simulink model "test"  (R2023b)
settings: Solver=FixedStepDiscrete  StartTime=0.0  StopTime=240  FixedStep=0.01  RelTol=1e-3
undefined symbols (not defined in the file or in its folder): DiscIntNeverNeededParam, InputPWM, WheelSpeed
libraries: mobileRoboticsTrainingLib x7, simulink x3
settings Model: SimulationMode=accelerator  NumberOfSteps=10  SnapshotBufferSize=20  Creator=Boitumelo  LastModifiedBy=kianf
settings DebuggingCC: UnconnectedInputMsg=warning  UnconnectedOutputMsg=warning  UnconnectedLineMsg=warning
settings ModelReferenceCC: EnableRefExpFcnMdlSchedulingChecks=on
settings RTWCC: DLArmComputeVersion=19.05

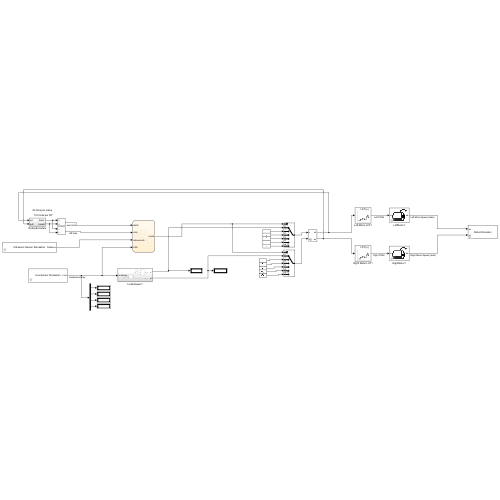
[thumbnail: Simulink's stored preview of the top-level diagram]
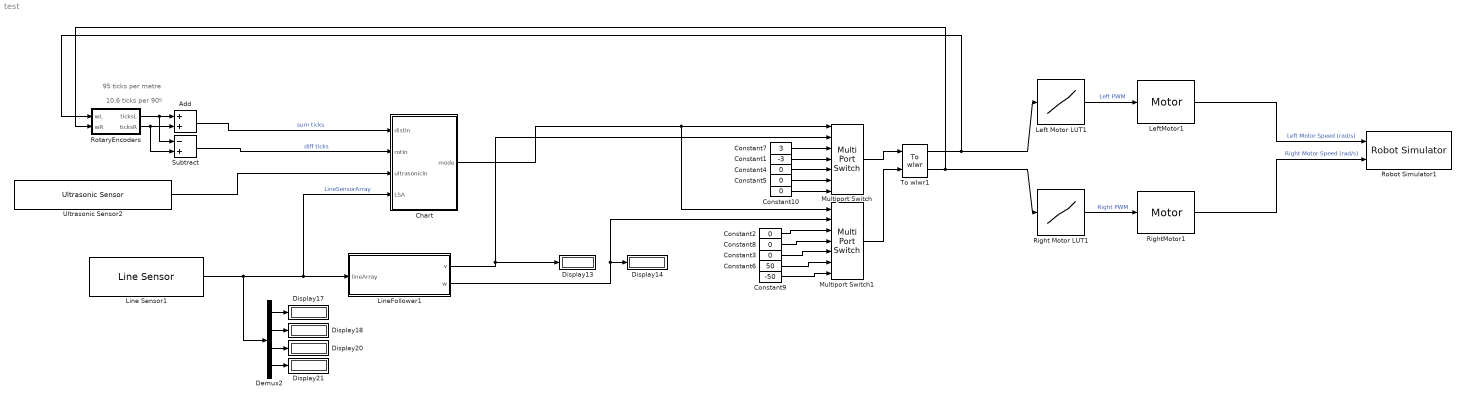
== system test ==
  note: 10.6 ticks per 90º
  note: 95 ticks per metre
  Add : Sum
  Chart : Stateflow chart  TreatAsAtomicUnit=on
  Constant1 : Constant  Value=-3
  Constant{2..5,8,10} (6 alike) : Constant  Value=0
  Constant6 : Constant  Value=50
  Constant7 : Constant  Value=3
  Constant9 : Constant  Value=-50
  Demux2 : Demux
  Display{13..14,17..18,20..21} (6 alike) : Display
  Left Motor LUT1 : Lookup_n-D  NumberOfTableDimensions=1  BreakpointsForDimension1=WheelSpeed  Table=InputPWM  InterpMethod=Nearest  ExtrapMethod=Clip  InternalRulePriority=Speed  RndMeth=Simplest
  LeftMotor1 : mobileRoboticsTrainingLib/Motor  motorPlant=wheelMotorModel  sensorType=Speed
      settings: SourceProductName=Mobile Robotics Training Library
  Line Sensor1 : mobileRoboticsTrainingLib/Line Sensor  mapVariable=mapForSim  envVal=1  lineVal=0  sensOff=[64.3e-3 35.4e-3;67.5e-3 5e-3;67.5e-3 -5e-3;64.3e-3 -35.4e-3]
      settings: SourceProductName=Mobile Robotics Training Library
  LineFollower1 : Subsystem
  Multiport Switch : MultiPortSwitch  DataPortOrder=Zero-based contiguous  Inputs=6  DataPortIndices={0,1,3,4}  zeroidx=on  SaturateOnIntegerOverflow=off
  Multiport Switch1 : MultiPortSwitch  DataPortOrder=Zero-based contiguous  Inputs=6  DataPortIndices={0,1,3,4}  zeroidx=on  SaturateOnIntegerOverflow=off  InputSameDT=off
  Right Motor LUT1 : Lookup_n-D  NumberOfTableDimensions=1  BreakpointsForDimension1=WheelSpeed  Table=InputPWM  InterpMethod=Nearest  ExtrapMethod=Clip  InternalRulePriority=Speed  RndMeth=Simplest
  RightMotor1 : mobileRoboticsTrainingLib/Motor  motorPlant=wheelMotorModel  sensorType=Speed
      settings: SourceProductName=Mobile Robotics Training Library
  Robot Simulator1 : mobileRoboticsTrainingLib/Robot Simulator  Priority=99  mapVar=mapForSim  startX=1  startY=0.27175  startTheta=90  axleLength=axleLength  wheelR=wheelR
  RotaryEncoders : Subsystem
  Subtract : Sum  Inputs=-+
  To wlwr1 : mobileRoboticsTrainingLib/To wlwr  axleLength=0.1  wheelR=0.05
      link override change parameters: Gain=[1 -axleLength/2;1 axleLength/2]
  Ultrasonic Sensor2 : mobileRoboticsTrainingLib/Ultrasonic Sensor  mapVar=mapForSim  maxSenRange=2  minSenRange=0.02  senRes=0.01  sensOff=[0 0]
      settings: SourceProductName=Mobile Robotics Training Library
  wires:
  RotaryEncoders/2(ticksR) -> Subtract/2, Add/2
  Ultrasonic Sensor2/1 -> Chart/3(ultrasonicIn)
  Demux2/3 -> Display20/1
  Demux2/2 -> Display18/1
  RotaryEncoders/1(ticksL) -> Subtract/1, Add/1
  Constant9/1 -> Multiport Switch1/7
  Add/1 -> Chart/1(distIn)  "sum ticks"
  Constant5/1 -> Multiport Switch/6
  Constant8/1 -> Multiport Switch1/4
  Multiport Switch/1 -> To wlwr1/1
  LineFollower1/2(w) -> Multiport Switch1/2, Display14/1
  Subtract/1 -> Chart/2(rotIn)  "diff ticks"
  Constant2/1 -> Multiport Switch1/3
  Demux2/4 -> Display21/1
  Constant1/1 -> Multiport Switch/4
  Constant4/1 -> Multiport Switch/5
  Demux2/1 -> Display17/1
  Constant7/1 -> Multiport Switch/3
  Constant3/1 -> Multiport Switch1/5
  Constant10/1 -> Multiport Switch/7
  Line Sensor1/1 -> Demux2/1, Chart/4(LSA), LineFollower1/1(lineArray)  "LineSensorArray"
  Constant6/1 -> Multiport Switch1/6
  Chart/1(mode) -> Multiport Switch1/1, Multiport Switch/1
  Multiport Switch1/1 -> To wlwr1/2
  LineFollower1/1(v) -> Display13/1, Multiport Switch/2
  LeftMotor1/1 -> Robot Simulator1/1  "Left Motor Speed (rad/s)"
  RightMotor1/1 -> Robot Simulator1/2  "Right Motor Speed (rad/s)"
  To wlwr1/1 -> RotaryEncoders/1(wL), Left Motor LUT1/1
  To wlwr1/2 -> Right Motor LUT1/1, RotaryEncoders/2(wR)
  Left Motor LUT1/1 -> LeftMotor1/1  "Left PWM"
  Right Motor LUT1/1 -> RightMotor1/1  "Right PWM"

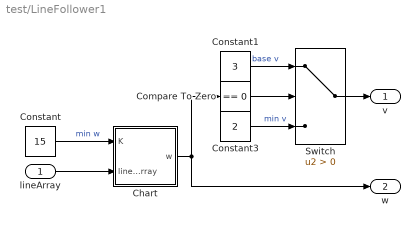
== system test/LineFollower1 ==
  lineArray : Inport
  Chart : Stateflow chart  TreatAsAtomicUnit=on
  Compare To Zero : simulink/Logic and Bit Operations/Compare To Zero  relop===  OutDataTypeStr=boolean
  Constant : Constant  Value=15
  Constant1 : Constant  Value=3
  Constant3 : Constant  Value=2
  Switch : Switch  Criteria=u2 > Threshold  SaturateOnIntegerOverflow=off  InputSameDT=off
  v : Outport
  w : Outport  Port=2
  wires:
  Constant1/1 -> Switch/1  "base v"
  Chart/1(w) -> Compare To Zero/1, w/1
  Constant3/1 -> Switch/3  "min v"
  Switch/1 -> v/1
  lineArray/1 -> Chart/2(lineArray)
  Compare To Zero/1 -> Switch/2
  Constant/1 -> Chart/1(K)  "min w"

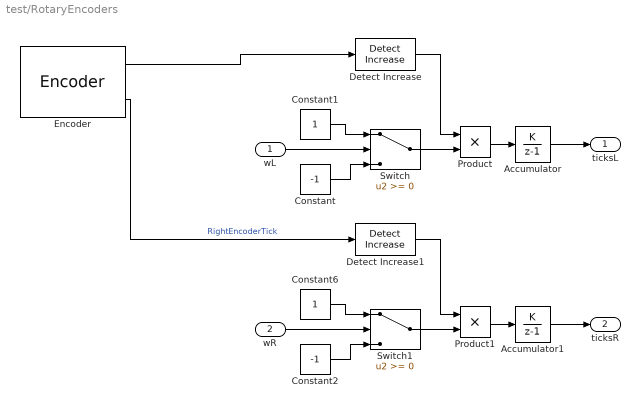
== system test/RotaryEncoders ==
  wL : Inport
  wR : Inport  Port=2
  Accumulator : DiscreteIntegrator  IntegratorMethod=Accumulation: Forward Euler  SampleTime=-1  ICPrevOutput=DiscIntNeverNeededParam  ICPrevScaledInput=DiscIntNeverNeededParam
  Accumulator1 : DiscreteIntegrator  IntegratorMethod=Accumulation: Forward Euler  SampleTime=-1  ICPrevOutput=DiscIntNeverNeededParam  ICPrevScaledInput=DiscIntNeverNeededParam
  Constant : Constant  Value=-1
  Constant1 : Constant
  Constant2 : Constant  Value=-1
  Constant6 : Constant
  Detect Increase : simulink/Logic and Bit Operations/Detect Increase  vinit=0.0  OutDataTypeStr=boolean
  Detect Increase1 : simulink/Logic and Bit Operations/Detect Increase  vinit=0.0  OutDataTypeStr=boolean
  Encoder : mobileRoboticsTrainingLib/Encoder  axleLength=axleLength  wheelR=wheelR  ticksPerRot=ticksPerRot
      settings: SourceProductName=Mobile Robotics Training Library
  Product : Product
  Product1 : Product
  Switch : Switch  SaturateOnIntegerOverflow=off  InputSameDT=off
  Switch1 : Switch  SaturateOnIntegerOverflow=off  InputSameDT=off
  ticksL : Outport
  ticksR : Outport  Port=2
  wires:
  wL/1 -> Switch/2
  Constant1/1 -> Switch/1
  Constant/1 -> Switch/3
  Encoder/1 -> Detect Increase/1
  Switch/1 -> Product/2
  Accumulator/1 -> ticksL/1
  wR/1 -> Switch1/2
  Constant6/1 -> Switch1/1
  Constant2/1 -> Switch1/3
  Accumulator1/1 -> ticksR/1
  Switch1/1 -> Product1/2
  Product/1 -> Accumulator/1
  Detect Increase/1 -> Product/1
  Detect Increase1/1 -> Product1/1
  Product1/1 -> Accumulator1/1
  Encoder/2 -> Detect Increase1/1  "RightEncoderTick"

== stateflow chart test/Chart ==
  state Setup
    entry:
    stop=0;
    objects = ones(5);
    object = 1;
  state Drive
    entry:
    mode=0;
  state DriveForward
    entry:
    mode = 1;
    distT = distIn + 8;
  state CentreOnIntersection
    entry:
    mode = 1;
    distT = distIn + 6;
  state LeftTurn
    entry:
    mode = 4;
    rotT = rotIn + 16;
  state RightTurn
    entry:
    mode = 5;
  state ErrorHandler
    entry:
    mode=4;
  state TurnAround
    entry:
    mode = 4;
    rotT = rotIn + 21;
  state ClosestObject
    entry:
    cObj = 1;
    for i = 1:5
    if objects(i) < cObj
    cObj = objects(i);
    end
    end
  state DriveBackward
    entry:
    mode = 2;
  state USmeasure
    entry:
    objects(object) = ultrasonicIn;
    object = object + 1;
  state Stop
    entry:
    mode=3;
  state Party
    state dance
      entry:
      moves = moves + 1;
    dance -> (junction 71) [order 2] : {mode=1;}
        | %1
    (junction 101) -> dance
    (junction 97) -> (junction 101) : after(125, msec)
    (junction 71) -> (junction 73) : after(250, msec)
        | {mode=2;}
        | %1+
    (junction 98) -> (junction 97) : after(125, msec)
        | {mode=3;}
        | %4a+d
    (junction 73) -> (junction 75) : after(250, msec)
        | {mode=4;}
        | %2
    (junction 75) -> (junction 76) : after(250, msec)
        | {mode=5;}
        | %2a+
    (junction 90) -> (junction 98) : after(250, msec)
        | {mode=5;}
        | %4a+
    (junction 76) -> (junction 77) : after(125, msec)
        | {mode=3;}
        | %2a+d
    (junction 85) -> (junction 90) : after(125, msec)
        | {mode=4;}
        | %4
    (junction 77) -> (junction 81) : after(125, msec)
        | {mode=4;}
        | %3
    (junction 81) -> (junction 91) : after(250, msec)
        | {mode=5;}
        | %3a+
    (junction 91) -> (junction 85) : after(125, msec)
        | {mode=3;}
        | %3a+d
  state Pause
    entry:
    mode=3;
    moves = 0;
  (default) -> Setup
  Setup -> Drive
  Drive -> TurnAround [order 2] : [all(LSA==1)]
  Drive -> (junction 8) [order 1] : [~LSA(1) | ~LSA(4)]{mode=3;}
  RightTurn -> Drive : [LSA(2)==0]
  TurnAround -> Drive : [rotIn>rotT]
  (junction 8) -> DriveForward [order 1] : [~LSA(1) & ~LSA(4)]
  (junction 8) -> CentreOnIntersection [order 2]
  CentreOnIntersection -> LeftTurn : [distIn>distT]
  LeftTurn -> RightTurn : [rotIn>rotT]
  DriveForward -> DriveBackward [order 2] : [LSA(1) & LSA(4)]
  DriveForward -> (junction 35) [order 1] : [distIn>distT]
      | {stop = stop + 1;}
  (junction 54) -> CentreOnIntersection [order 2]
  (junction 35) -> ErrorHandler [order 2] : [stop>2]
  (junction 35) -> (junction 63) [order 3]
  (junction 63) -> TurnAround
  ClosestObject -> (junction 63)
  (junction 57) -> (junction 63) [order 2]
  (junction 35) -> ClosestObject [order 1] : [stop==2]
  USmeasure -> (junction 63)
  DriveBackward -> (junction 54) : [~LSA(1) & ~LSA(4)]
      | {mode=3}
  (junction 54) -> (junction 141) [order 1] : [ultrasonicIn & (ultrasonicIn < 0.5)]
  (junction 141) -> USmeasure [order 2]
  (junction 141) -> (junction 57) [order 1] : [stop==2]
  dance -> Stop [order 1] : [moves > 4]
  (junction 57) -> Pause [order 1] : [abs(ultrasonicIn-cObj) <= 0.03]
  Pause -> (junction 71) : after(3,sec)
      | {mode=1;}
      | %1
  data: distIn input; rotIn input; mode output; ultrasonicIn input; LSA input; distT local; rotT local; objects local; stop local; cObj local; i local; object local; moves local

== stateflow chart test/LineFollower1/Chart ==
  state ComputeW
    %code for the line array
    during:
    w = K*(lineArray(3)-lineArray(2));
  (default) -> ComputeW
  data: w output; K input; lineArray input
